simulink model "PID_outer"  (R2022a)
settings: Solver=FixedStepAuto  StartTime=0.0  StopTime=T  FixedStep=Ts  RelTol=1e-3
values from neighbouring files (symbols this model uses):
  den_c = [0.0176838825658 1 0]    [matlab.mat]
  den_d = [1 -2.9359258401 2.87204282074 -0.936116980647]    [matlab.mat]
  freq_w = 1.0471975512    [matlab.mat]    (also in outerloop_design_simulation.m = 1.25663706144)
  Kd = -1.25238088599    [matlab.mat]    (also in outerloop_design_simulation.m = -0.5)
  Ki = -0.366174642792    [matlab.mat]    (also in outerloop_design_simulation.m = -0.25)
  Kp = -2.30865925239    [matlab.mat]    (also in outerloop_design_simulation.m = -0.3)
  N = 171.428571429    [matlab.mat]    (also in outerloop_design_simulation.m = 3.1722)
  num_c = [-3.02394391875 -20.9 -11.9380520836]    [matlab.mat]
  num_d = [-0.152140650499 0.152068965288 0.152140642993 -0.152068972794]    [matlab.mat]
  radius = 0    [matlab.mat]    (also in outerloop_design_simulation.m = 0.1)
  sat_lb = -0.0872664625997    [matlab.mat]    (also in outerloop_design_simulation.m)
  sat_ub = 0.0872664625997    [matlab.mat]    (also in outerloop_design_simulation.m)
  sys_den = [1 0 0]    [matlab.mat]    (also in outerloop_design_simulation.m = sys_tf1.den{:})
  sys_num = [0 0 -7.00714285714]    [matlab.mat]    (also in outerloop_design_simulation.m = sys_tf1.num{:})
  Ts = 0.035    [matlab.mat]    (also in outerloop_design_simulation.m)
libraries: simulink_extras x8, slpidlib x4
settings Model: Creator=michi  LastModifiedBy=michi

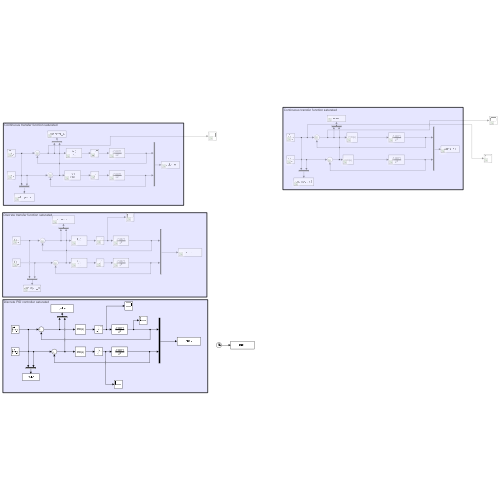
[thumbnail: Simulink's stored preview of the top-level diagram]
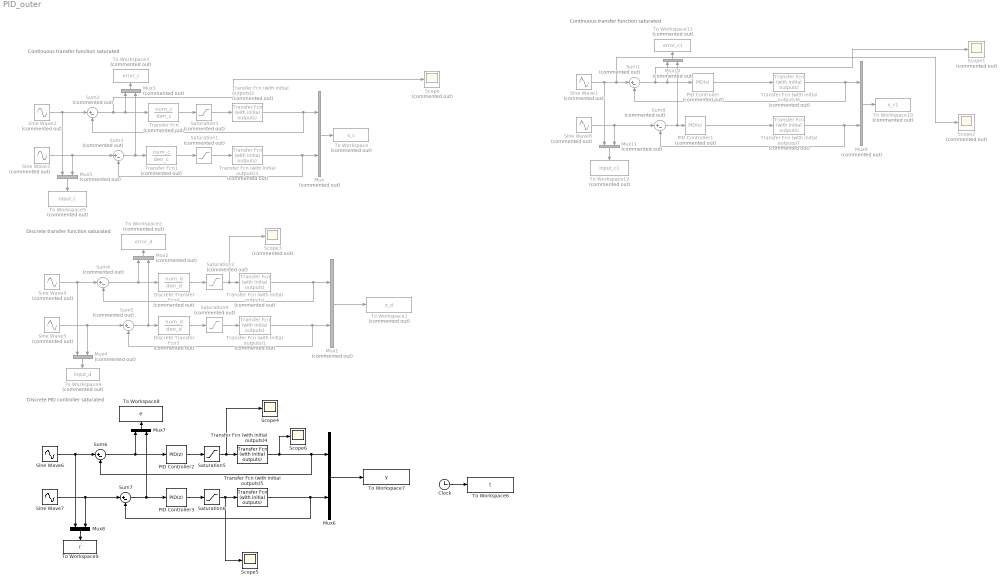
== system PID_outer ==
  note: Discrete PID controller saturated
  note: Discrete transfer function saturated
  note: Continuous transfer function saturated
  note: Continuous transfer function saturated
  Clock : Clock
  Discrete Transfer Fcn3 : DiscreteTransferFcn  Commented=on  Numerator=num_d  Denominator=den_d  SampleTime=Ts
  Discrete Transfer Fcn4 : DiscreteTransferFcn  Commented=on  Numerator=num_d  Denominator=den_d  SampleTime=Ts
  Mux{,1..5,9..11} (9 alike) : Mux  Commented=on  Inputs=2
  Mux6 : Mux  Inputs=2
  Mux7 : Mux  Inputs=2
  Mux8 : Mux  Inputs=2
  PID Controller : slpidlib/PID Controller  Commented=on  Controller=PID  Form=Parallel  TimeDomain=Continuous-time  UseExternalTs=off  SampleTime=-1  IntegratorMethod=Forward Euler  FilterMethod=Forward Euler  ControllerParametersSource=internal  P=-0.0265  I=-0.00124  UseKiTs=off  D=-0.139  N=1/0.183  UseFilter=on  TunerSelectOption=Transfer Function Based (PID Tuner App)  InitialConditionSource=internal  InitialConditionForIntegrator=0  InitialConditionForFilter=0  DifferentiatorICPrevScaledInput=0  ExternalReset=none  TrackingMode=off  Kt=1  LimitOutput=off  SatLimitsSource=internal  UpperSaturationLimit=inf  LowerSaturationLimit=-inf  LinearizeAsGain=on  AntiWindupMode=none  Kb=1  POutMin=[]  POutMax=[]  IOutMin=[]  IOutMax=[]  DOutMin=[]  DOutMax=[]  NOutMin=[]  NOutMax=[]  SumOutMin=[]  SumOutMax=[]  SaturationOutMin=[]  SaturationOutMax=[]  PParamMin=[]  PParamMax=[]  IParamMin=[]  IParamMax=[]  DParamMin=[]  DParamMax=[]  NParamMin=[]  NParamMax=[]  KbParamMin=[]  KbParamMax=[]  KtParamMin=[]  KtParamMax=[]  KbOutMin=[]  KbOutMax=[]  KtOutMin=[]  KtOutMax=[]  IntegratorOutMin=[]  IntegratorOutMax=[]  FilterOutMin=[]  FilterOutMax=[]  SumI1OutMin=[]  SumI1OutMax=[]  SumI2OutMin=[]  SumI2OutMax=[]  SumI3OutMin=[]  SumI3OutMax=[]  SumI4OutMin=[]  SumI4OutMax=[]  SumDOutMin=[]  SumDOutMax=[]  DifferentiatorOutMin=[]  DifferentiatorOutMax=[]  FilterDiffOutCoefMin=[]  FilterDiffOutCoefMax=[]  ReciprocalOutMin=[]  ReciprocalOutMax=[]  SumDenOutMin=[]  SumDenOutMax=[]  SumNumOutMin=[]  SumNumOutMax=[]  DivideOutMin=[]  DivideOutMax=[]  UdiffTsProdOutMin=[]  UdiffTsProdOutMax=[]  NTsProdOutMin=[]  NTsProdOutMax=[]  UintegralTsProdOutMin=[]  UintegralTsProdOutMax=[]  UngainTsProdOutMin=[]  UngainTsProdOutMax=[]  IntegratorContinuousStateAttributes=''  IntegratorStateMustResolveToSignalObject=off  IntegratorRTWStateStorageClass=Auto  FilterContinuousStateAttributes=''  FilterStateMustResolveToSignalObject=off  FilterRTWStateStorageClass=Auto  ParallelPVariant=InternalParameters  IdealPVariant=Disabled  IVariant=InternalParameters  DVariant=InternalParameters  IntegratorVariant=Continuous  SatVariant=Disabled  AWVariant=Passthrough  PCopyVariant=Disabled  TRVariant=Disabled  FdbkBlocksVariant=Forward  IdealPFdbkVariant=Disabled  SatFdbkVariant=Disabled  DerivativeFilterVariant=ContFilter  NVariant=InternalParameters  NCopyVariant=Disabled  FilterICVariant=InternalICsFilter  IntegratorICVariant=InternalICs  ExternalResetVariant=Disabled  TRSumVariant=Passthrough  SumFdbkVariant=Disabled  SumVariant=Sum_PID  TsampFilterVariant=InternalTs  TsampNgainVariant=Passthrough  TsampIntegralVariant=Passthrough  ExternalSaturationOutDataTypeStr=Inherit: Same as second input  aMode=0
  PID Controller1 : slpidlib/PID Controller  Commented=on  Controller=PID  Form=Parallel  TimeDomain=Continuous-time  UseExternalTs=off  SampleTime=-1  IntegratorMethod=Forward Euler  FilterMethod=Forward Euler  ControllerParametersSource=internal  P=-0.0265  I=-0.00124  UseKiTs=off  D=-0.139  N=1/0.183  UseFilter=on  TunerSelectOption=Transfer Function Based (PID Tuner App)  InitialConditionSource=internal  InitialConditionForIntegrator=0  InitialConditionForFilter=0  DifferentiatorICPrevScaledInput=0  ExternalReset=none  TrackingMode=off  Kt=1  LimitOutput=off  SatLimitsSource=internal  UpperSaturationLimit=inf  LowerSaturationLimit=-inf  LinearizeAsGain=on  AntiWindupMode=none  Kb=1  POutMin=[]  POutMax=[]  IOutMin=[]  IOutMax=[]  DOutMin=[]  DOutMax=[]  NOutMin=[]  NOutMax=[]  SumOutMin=[]  SumOutMax=[]  SaturationOutMin=[]  SaturationOutMax=[]  PParamMin=[]  PParamMax=[]  IParamMin=[]  IParamMax=[]  DParamMin=[]  DParamMax=[]  NParamMin=[]  NParamMax=[]  KbParamMin=[]  KbParamMax=[]  KtParamMin=[]  KtParamMax=[]  KbOutMin=[]  KbOutMax=[]  KtOutMin=[]  KtOutMax=[]  IntegratorOutMin=[]  IntegratorOutMax=[]  FilterOutMin=[]  FilterOutMax=[]  SumI1OutMin=[]  SumI1OutMax=[]  SumI2OutMin=[]  SumI2OutMax=[]  SumI3OutMin=[]  SumI3OutMax=[]  SumI4OutMin=[]  SumI4OutMax=[]  SumDOutMin=[]  SumDOutMax=[]  DifferentiatorOutMin=[]  DifferentiatorOutMax=[]  FilterDiffOutCoefMin=[]  FilterDiffOutCoefMax=[]  ReciprocalOutMin=[]  ReciprocalOutMax=[]  SumDenOutMin=[]  SumDenOutMax=[]  SumNumOutMin=[]  SumNumOutMax=[]  DivideOutMin=[]  DivideOutMax=[]  UdiffTsProdOutMin=[]  UdiffTsProdOutMax=[]  NTsProdOutMin=[]  NTsProdOutMax=[]  UintegralTsProdOutMin=[]  UintegralTsProdOutMax=[]  UngainTsProdOutMin=[]  UngainTsProdOutMax=[]  IntegratorContinuousStateAttributes=''  IntegratorStateMustResolveToSignalObject=off  IntegratorRTWStateStorageClass=Auto  FilterContinuousStateAttributes=''  FilterStateMustResolveToSignalObject=off  FilterRTWStateStorageClass=Auto  ParallelPVariant=InternalParameters  IdealPVariant=Disabled  IVariant=InternalParameters  DVariant=InternalParameters  IntegratorVariant=Continuous  SatVariant=Disabled  AWVariant=Passthrough  PCopyVariant=Disabled  TRVariant=Disabled  FdbkBlocksVariant=Forward  IdealPFdbkVariant=Disabled  SatFdbkVariant=Disabled  DerivativeFilterVariant=ContFilter  NVariant=InternalParameters  NCopyVariant=Disabled  FilterICVariant=InternalICsFilter  IntegratorICVariant=InternalICs  ExternalResetVariant=Disabled  TRSumVariant=Passthrough  SumFdbkVariant=Disabled  SumVariant=Sum_PID  TsampFilterVariant=InternalTs  TsampNgainVariant=Passthrough  TsampIntegralVariant=Passthrough  ExternalSaturationOutDataTypeStr=Inherit: Same as second input  aMode=0
  PID Controller2 : slpidlib/PID Controller  Controller=PID  Form=Parallel  TimeDomain=Discrete-time  UseExternalTs=off  SampleTime=Ts  IntegratorMethod=Forward Euler  FilterMethod=Forward Euler  ControllerParametersSource=internal  P=Kp  I=Ki  UseKiTs=off  D=Kd  N=N  UseFilter=on  TunerSelectOption=Transfer Function Based (PID Tuner App)  InitialConditionSource=internal  InitialConditionForIntegrator=0  InitialConditionForFilter=0  DifferentiatorICPrevScaledInput=0  ExternalReset=none  TrackingMode=off  Kt=1  LimitOutput=off  SatLimitsSource=internal  UpperSaturationLimit=inf  LowerSaturationLimit=-inf  LinearizeAsGain=on  AntiWindupMode=none  Kb=1  POutMin=[]  POutMax=[]  IOutMin=[]  IOutMax=[]  DOutMin=[]  DOutMax=[]  NOutMin=[]  NOutMax=[]  SumOutMin=[]  SumOutMax=[]  SaturationOutMin=[]  SaturationOutMax=[]  PParamMin=[]  PParamMax=[]  IParamMin=[]  IParamMax=[]  DParamMin=[]  DParamMax=[]  NParamMin=[]  NParamMax=[]  KbParamMin=[]  KbParamMax=[]  KtParamMin=[]  KtParamMax=[]  KbOutMin=[]  KbOutMax=[]  KtOutMin=[]  KtOutMax=[]  IntegratorOutMin=[]  IntegratorOutMax=[]  FilterOutMin=[]  FilterOutMax=[]  SumI1OutMin=[]  SumI1OutMax=[]  SumI2OutMin=[]  SumI2OutMax=[]  SumI3OutMin=[]  SumI3OutMax=[]  SumI4OutMin=[]  SumI4OutMax=[]  SumDOutMin=[]  SumDOutMax=[]  DifferentiatorOutMin=[]  DifferentiatorOutMax=[]  FilterDiffOutCoefMin=[]  FilterDiffOutCoefMax=[]  ReciprocalOutMin=[]  ReciprocalOutMax=[]  SumDenOutMin=[]  SumDenOutMax=[]  SumNumOutMin=[]  SumNumOutMax=[]  DivideOutMin=[]  DivideOutMax=[]  UdiffTsProdOutMin=[]  UdiffTsProdOutMax=[]  NTsProdOutMin=[]  NTsProdOutMax=[]  UintegralTsProdOutMin=[]  UintegralTsProdOutMax=[]  UngainTsProdOutMin=[]  UngainTsProdOutMax=[]  IntegratorContinuousStateAttributes=''  IntegratorStateMustResolveToSignalObject=off  IntegratorRTWStateStorageClass=Auto  FilterContinuousStateAttributes=''  FilterStateMustResolveToSignalObject=off  FilterRTWStateStorageClass=Auto  ParallelPVariant=InternalParameters  IdealPVariant=Disabled  IVariant=InternalParameters  DVariant=InternalParameters  IntegratorVariant=Discrete  SatVariant=Disabled  AWVariant=Passthrough  PCopyVariant=Disabled  TRVariant=Disabled  FdbkBlocksVariant=Forward  IdealPFdbkVariant=Disabled  SatFdbkVariant=Disabled  DerivativeFilterVariant=ForwardEulerFilter  NVariant=InternalParameters  NCopyVariant=Disabled  FilterICVariant=InternalICsFilter  IntegratorICVariant=InternalICs  ExternalResetVariant=Disabled  TRSumVariant=Passthrough  SumFdbkVariant=Disabled  SumVariant=Sum_PID  TsampFilterVariant=InternalTs  TsampNgainVariant=Passthrough  TsampIntegralVariant=Passthrough  ExternalSaturationOutDataTypeStr=Inherit: Same as second input  aMode=0
  PID Controller3 : slpidlib/PID Controller  Controller=PID  Form=Parallel  TimeDomain=Discrete-time  UseExternalTs=off  SampleTime=Ts  IntegratorMethod=Forward Euler  FilterMethod=Forward Euler  ControllerParametersSource=internal  P=Kp  I=Ki  UseKiTs=off  D=Kd  N=N  UseFilter=on  TunerSelectOption=Transfer Function Based (PID Tuner App)  InitialConditionSource=internal  InitialConditionForIntegrator=0  InitialConditionForFilter=0  DifferentiatorICPrevScaledInput=0  ExternalReset=none  TrackingMode=off  Kt=1  LimitOutput=off  SatLimitsSource=internal  UpperSaturationLimit=inf  LowerSaturationLimit=-inf  LinearizeAsGain=on  AntiWindupMode=none  Kb=1  POutMin=[]  POutMax=[]  IOutMin=[]  IOutMax=[]  DOutMin=[]  DOutMax=[]  NOutMin=[]  NOutMax=[]  SumOutMin=[]  SumOutMax=[]  SaturationOutMin=[]  SaturationOutMax=[]  PParamMin=[]  PParamMax=[]  IParamMin=[]  IParamMax=[]  DParamMin=[]  DParamMax=[]  NParamMin=[]  NParamMax=[]  KbParamMin=[]  KbParamMax=[]  KtParamMin=[]  KtParamMax=[]  KbOutMin=[]  KbOutMax=[]  KtOutMin=[]  KtOutMax=[]  IntegratorOutMin=[]  IntegratorOutMax=[]  FilterOutMin=[]  FilterOutMax=[]  SumI1OutMin=[]  SumI1OutMax=[]  SumI2OutMin=[]  SumI2OutMax=[]  SumI3OutMin=[]  SumI3OutMax=[]  SumI4OutMin=[]  SumI4OutMax=[]  SumDOutMin=[]  SumDOutMax=[]  DifferentiatorOutMin=[]  DifferentiatorOutMax=[]  FilterDiffOutCoefMin=[]  FilterDiffOutCoefMax=[]  ReciprocalOutMin=[]  ReciprocalOutMax=[]  SumDenOutMin=[]  SumDenOutMax=[]  SumNumOutMin=[]  SumNumOutMax=[]  DivideOutMin=[]  DivideOutMax=[]  UdiffTsProdOutMin=[]  UdiffTsProdOutMax=[]  NTsProdOutMin=[]  NTsProdOutMax=[]  UintegralTsProdOutMin=[]  UintegralTsProdOutMax=[]  UngainTsProdOutMin=[]  UngainTsProdOutMax=[]  IntegratorContinuousStateAttributes=''  IntegratorStateMustResolveToSignalObject=off  IntegratorRTWStateStorageClass=Auto  FilterContinuousStateAttributes=''  FilterStateMustResolveToSignalObject=off  FilterRTWStateStorageClass=Auto  ParallelPVariant=InternalParameters  IdealPVariant=Disabled  IVariant=InternalParameters  DVariant=InternalParameters  IntegratorVariant=Discrete  SatVariant=Disabled  AWVariant=Passthrough  PCopyVariant=Disabled  TRVariant=Disabled  FdbkBlocksVariant=Forward  IdealPFdbkVariant=Disabled  SatFdbkVariant=Disabled  DerivativeFilterVariant=ForwardEulerFilter  NVariant=InternalParameters  NCopyVariant=Disabled  FilterICVariant=InternalICsFilter  IntegratorICVariant=InternalICs  ExternalResetVariant=Disabled  TRSumVariant=Passthrough  SumFdbkVariant=Disabled  SumVariant=Sum_PID  TsampFilterVariant=InternalTs  TsampNgainVariant=Passthrough  TsampIntegralVariant=Passthrough  ExternalSaturationOutDataTypeStr=Inherit: Same as second input  aMode=0
  Saturation{1..4} (4 alike) : Saturate  Commented=on  UpperLimit=sat_ub  LowerLimit=sat_lb
  Saturation5 : Saturate  UpperLimit=sat_ub  LowerLimit=sat_lb
  Saturation6 : Saturate  UpperLimit=sat_ub  LowerLimit=sat_lb
  Scope{,1..3} (4 alike) : Scope  Commented=on
  Scope4 : Scope
  Scope5 : Scope
  Scope6 : Scope
  Sine Wave1 : Sin  Commented=on  Amplitude=0.1  Frequency=freq_w  Phase=pi/2  SampleTime=0
  Sine Wave2 : Sin  Commented=on  Amplitude=radius  Frequency=freq_w  Phase=pi/2  SampleTime=0
  Sine Wave3 : Sin  Commented=on  Amplitude=radius  Frequency=freq_w  SampleTime=0
  Sine Wave4 : Sin  Commented=on  Amplitude=radius  Frequency=freq_w  Phase=pi/2  SampleTime=Ts
  Sine Wave5 : Sin  Commented=on  Amplitude=radius  Frequency=freq_w  SampleTime=Ts
  Sine Wave6 : Sin  Amplitude=radius  Frequency=freq_w  Phase=pi/2  SampleTime=Ts
  Sine Wave7 : Sin  Amplitude=radius  Frequency=freq_w  SampleTime=Ts
  Sine Wave8 : Sin  Commented=on  Amplitude=0.1  Frequency=freq_w  SampleTime=0
  Sum{1..5,8} (6 alike) : Sum  Commented=on  Inputs=|+-
  Sum6 : Sum  Inputs=|+-
  Sum7 : Sum  Inputs=|+-
  To Workspace : ToWorkspace  Commented=on  VariableName=x_c  SampleTime=-1
  To Workspace1 : ToWorkspace  Commented=on  VariableName=x_d  SampleTime=-1
  To Workspace10 : ToWorkspace  Commented=on  VariableName=x_c1  SampleTime=-1
  To Workspace11 : ToWorkspace  Commented=on  VariableName=error_c1  SampleTime=-1
  To Workspace12 : ToWorkspace  Commented=on  VariableName=input_c1  SampleTime=-1
  To Workspace2 : ToWorkspace  Commented=on  VariableName=error_d  SampleTime=-1
  To Workspace3 : ToWorkspace  Commented=on  VariableName=error_c  SampleTime=-1
  To Workspace4 : ToWorkspace  Commented=on  VariableName=input_d  SampleTime=-1
  To Workspace5 : ToWorkspace  Commented=on  VariableName=input_c  SampleTime=-1
  To Workspace6 : ToWorkspace  VariableName=t  SampleTime=-1
  To Workspace7 : ToWorkspace  VariableName=y  SampleTime=-1
  To Workspace8 : ToWorkspace  VariableName=e  SampleTime=-1
  To Workspace9 : ToWorkspace  VariableName=r  SampleTime=-1
  Transfer Fcn : TransferFcn  Commented=on  Numerator=num_c  Denominator=den_c
  Transfer Fcn (with initial outputs) : simulink_extras/Additional Linear/Transfer Fcn (with initial outputs)  Commented=on  N=sys_num  D=sys_den  Y0=init_x  U0=0
  Transfer Fcn (with initial outputs)1 : simulink_extras/Additional Linear/Transfer Fcn (with initial outputs)  Commented=on  N=sys_num  D=sys_den  Y0=init_y  U0=0
  Transfer Fcn (with initial outputs)2 : simulink_extras/Additional Linear/Transfer Fcn (with initial outputs)  Commented=on  N=sys_num  D=sys_den  Y0=init_x  U0=0
  Transfer Fcn (with initial outputs)3 : simulink_extras/Additional Linear/Transfer Fcn (with initial outputs)  Commented=on  N=sys_num  D=sys_den  Y0=init_y  U0=0
  Transfer Fcn (with initial outputs)4 : simulink_extras/Additional Linear/Transfer Fcn (with initial outputs)  N=sys_num  D=sys_den  Y0=init_x  U0=0
  Transfer Fcn (with initial outputs)5 : simulink_extras/Additional Linear/Transfer Fcn (with initial outputs)  N=sys_num  D=sys_den  Y0=init_y  U0=0
  Transfer Fcn (with initial outputs)6 : simulink_extras/Additional Linear/Transfer Fcn (with initial outputs)  Commented=on  N=sys_num  D=sys_den  Y0=init_x  U0=0
  Transfer Fcn (with initial outputs)7 : simulink_extras/Additional Linear/Transfer Fcn (with initial outputs)  Commented=on  N=sys_num  D=sys_den  Y0=init_y  U0=0
  Transfer Fcn1 : TransferFcn  Commented=on  Numerator=num_c  Denominator=den_c
  wires:
  Mux/1 -> To Workspace/1
  Mux1/1 -> To Workspace1/1
  Sine Wave4/1 -> Sum4/1, Mux4/1
  Sine Wave5/1 -> Sum5/1, Mux4/2
  Sum4/1 -> Discrete Transfer Fcn4/1, Mux2/1
  Transfer Fcn (with initial outputs)/1 -> Sum4/2, Mux1/1
  Transfer Fcn (with initial outputs)1/1 -> Sum5/2, Mux1/2
  Sum5/1 -> Discrete Transfer Fcn3/1, Mux2/2
  Mux2/1 -> To Workspace2/1
  Discrete Transfer Fcn3/1 -> Saturation4/1
  Sum3/1 -> Transfer Fcn1/1, Mux3/2
  Mux3/1 -> To Workspace3/1
  Sum2/1 -> Scope/1, Transfer Fcn/1, Mux3/1
  Transfer Fcn (with initial outputs)2/1 -> Sum2/2, Mux/1
  Transfer Fcn (with initial outputs)3/1 -> Sum3/2, Mux/2
  Mux4/1 -> To Workspace4/1
  Discrete Transfer Fcn4/1 -> Saturation2/1
  Transfer Fcn/1 -> Saturation3/1
  Transfer Fcn1/1 -> Saturation1/1
  Sine Wave3/1 -> Sum3/1, Mux5/2
  Mux5/1 -> To Workspace5/1
  Sine Wave2/1 -> Sum2/1, Mux5/1
  Clock/1 -> To Workspace6/1
  Saturation2/1 -> Scope3/1, Transfer Fcn (with initial outputs)/1
  Saturation4/1 -> Transfer Fcn (with initial outputs)1/1
  Saturation1/1 -> Transfer Fcn (with initial outputs)3/1
  Saturation3/1 -> Transfer Fcn (with initial outputs)2/1
  Saturation5/1 -> Scope4/1, Transfer Fcn (with initial outputs)4/1
  PID Controller2/1 -> Saturation5/1
  Mux8/1 -> To Workspace9/1
  Sum6/1 -> PID Controller2/1, Mux7/1
  Sum7/1 -> PID Controller3/1, Mux7/2
  Mux7/1 -> To Workspace8/1
  Sine Wave6/1 -> Sum6/1, Mux8/1
  Sine Wave7/1 -> Sum7/1, Mux8/2
  Transfer Fcn (with initial outputs)4/1 -> Sum6/2, Mux6/1, Scope6/1
  Mux6/1 -> To Workspace7/1
  Saturation6/1 -> Scope5/1, Transfer Fcn (with initial outputs)5/1
  Transfer Fcn (with initial outputs)5/1 -> Sum7/2, Mux6/2
  PID Controller3/1 -> Saturation6/1
  Sine Wave8/1 -> Sum8/1, Mux11/2
  Sum8/1 -> PID Controller1/1, Mux10/2
  Transfer Fcn (with initial outputs)6/1 -> Sum1/2, Mux9/1
  PID Controller/1 -> Transfer Fcn (with initial outputs)6/1
  Sum1/1 -> Scope1/1, PID Controller/1, Mux10/1
  PID Controller1/1 -> Transfer Fcn (with initial outputs)7/1
  Mux10/1 -> To Workspace11/1
  Sine Wave1/1 -> Scope2/1, Sum1/1, Mux11/1
  Transfer Fcn (with initial outputs)7/1 -> Sum8/2, Mux9/2
  Mux11/1 -> To Workspace12/1
  Mux9/1 -> To Workspace10/1
